simulink subsystem "Send_GCS_Data_Fixed_Wing"  (R2025a)
settings: Solver=VariableStepAuto  StartTime=0.0  StopTime=10.0  RelTol=1e-3
libraries: px4uORBlib x2
settings Model: Creator=gurt1  LastModifiedBy=gurt1

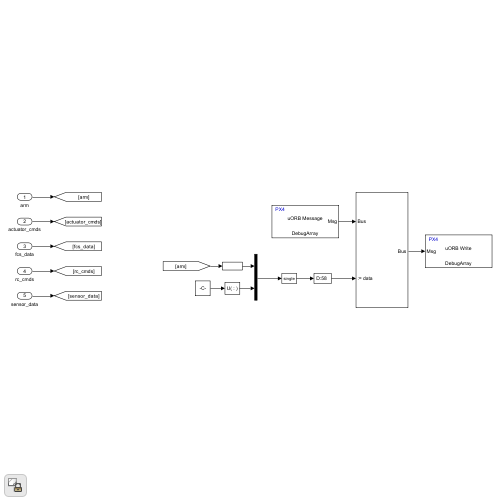
[thumbnail: Simulink's stored preview of the top-level diagram]
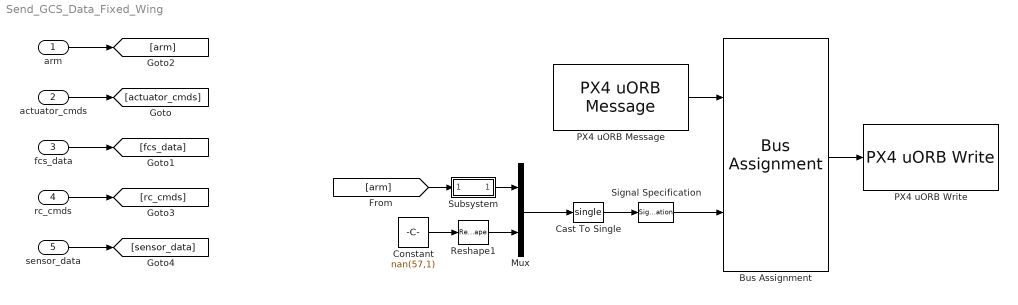
== system Send_GCS_Data_Fixed_Wing ==
  arm : Inport
  actuator_cmds : Inport  Port=2
  fcs_data : Inport  Port=3
  rc_cmds : Inport  Port=4
  sensor_data : Inport  Port=5
  Bus Assignment : BusAssignment  AssignedSignals=data
  Cast To Single : DataTypeConversion  OutDataTypeStr=single  SaturateOnIntegerOverflow=off  RndMeth=Floor
  Constant : Constant  Value=nan(57,1)
  Mux : Mux  Inputs=2
  PX4 uORB Message : px4uORBlib/PX4 uORB Message  uORBTopic=DebugArray  SampleTime=-1  selectInstance=DebugArray
  PX4 uORB Write : px4uORBlib/PX4 uORB Write  uORBTopic=DebugArray  selectInstance=DebugArray  MessageQueueLen=1
  Reshape1 : Reshape
  Signal Specification : SignalSpecification  Dimensions=58
  Subsystem : Subsystem
  wires:
  Reshape1/1 -> Mux/2
  Signal Specification/1 -> Bus Assignment/2
  Cast To Single/1 -> Signal Specification/1
  actuator_cmds/1 -> [actuator_cmds]
  Bus Assignment/1 -> PX4 uORB Write/1
  PX4 uORB Message/1 -> Bus Assignment/1
  arm/1 -> [arm]
  rc_cmds/1 -> [rc_cmds]
  Mux/1 -> Cast To Single/1
  sensor_data/1 -> [sensor_data]
  fcs_data/1 -> [fcs_data]
  Constant/1 -> Reshape1/1
  [arm] -> Subsystem/1(" ")
  Subsystem/1("  ") -> Mux/1

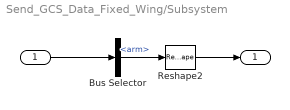
== system Send_GCS_Data_Fixed_Wing/Subsystem ==
  " " : Inport
  Bus Selector : BusSelector  OutputSignals=arm
  Reshape2 : Reshape
  "  " : Outport
  wires:
  Bus Selector/1 -> Reshape2/1  "<arm>"
  Reshape2/1 -> "  "/1
  " "/1 -> Bus Selector/1
